simulink model "ADC"  (R2024b)
settings: Solver=ode4  StartTime=0.0  StopTime=0.001  FixedStep=1e-6  RelTol=1e-3
undefined symbols (not defined in the file): DiscIntNeverNeededParam
settings Model: Creator=Asus  LastModifiedBy=Asus

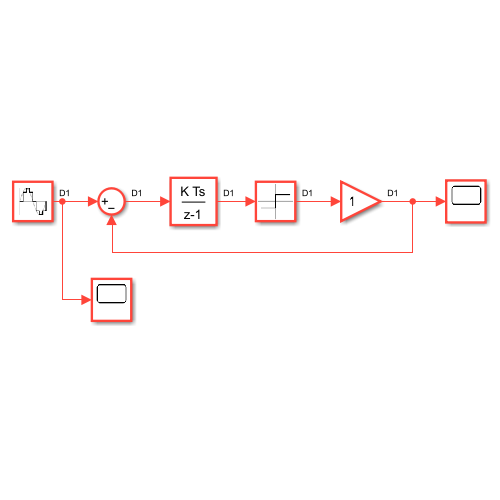
[thumbnail: Simulink's stored preview of the top-level diagram]
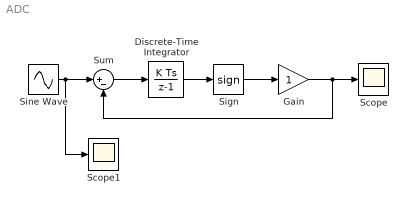
== system ADC ==
  Discrete-Time Integrator : DiscreteIntegrator  SampleTime=1e-6  ICPrevOutput=DiscIntNeverNeededParam  ICPrevScaledInput=DiscIntNeverNeededParam
  Gain : Gain
  Scope : Scope
  Scope1 : Scope
  Sign : Signum
  Sine Wave : Sin  Frequency=6283.1853  SampleTime=1e-6
  Sum : Sum  Inputs=|+-
  wires:
  Sine Wave/1 -> Scope1/1, Sum/1
  Sum/1 -> Discrete-Time Integrator/1
  Discrete-Time Integrator/1 -> Sign/1
  Gain/1 -> Scope/1, Sum/2
  Sign/1 -> Gain/1
